simulink subsystem "ACS"  (R2025a)
settings: Solver=VariableStepAuto  StartTime=0.0  StopTime=10.0  RelTol=1e-3
settings Model: Creator=Глеб  LastModifiedBy=Глеб

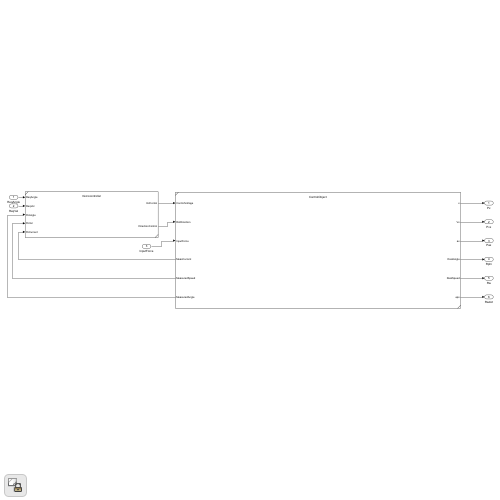
[thumbnail: Simulink's stored preview of the top-level diagram]
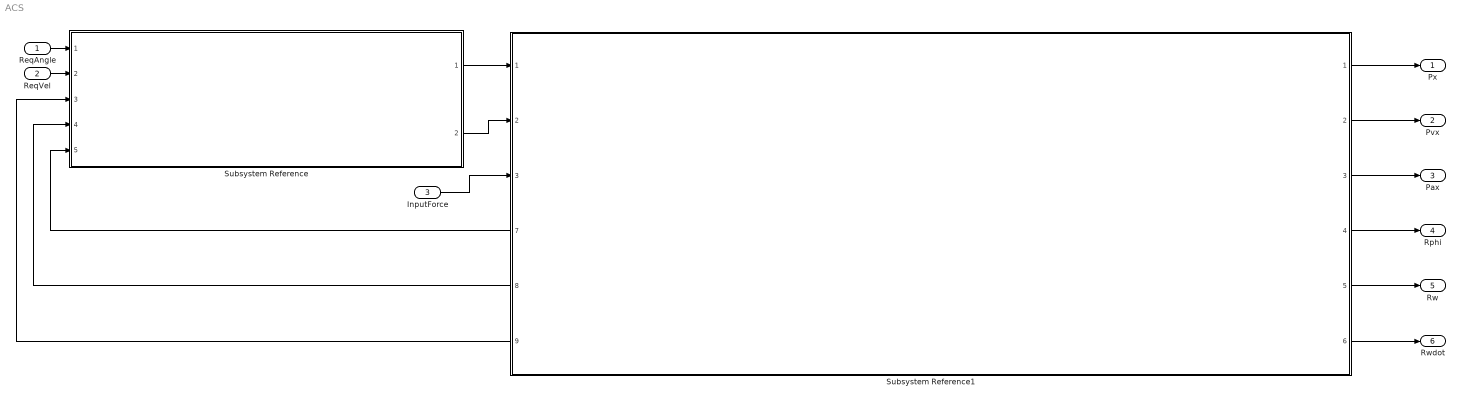
== system ACS ==
  ReqAngle : Inport
  ReqVel : Inport  Port=2
  InputForce : Inport  Port=3
  Subsystem Reference : Subsystem  ReferencedSubsystem=microcontroller
  Subsystem Reference1 : Subsystem  ReferencedSubsystem=ControlObject
      settings: PortSchema="{\"entries\":[{\"content\":{\"sides\":[{\"content\":{\"connectorIds\":[\"In1\",\"In2\",\"In3\",\"Out7\",\"Out8\",\"Out9\"]},\"type\":\"ConnectorPlacement.EquallySpacedRectSide\",\"uuid\":\"186974e8-f72a-4b37-bad7-12b1ef69ccf2\"},{\"content\":{\"connectorIds\":[\"Out1\",\"Out2\",\"Out3\",\"Out4\",\"Out5\",\"Out6\"],\"side\":\"RIGHT\"},\"type\":\"ConnectorPlacement.EquallySpacedRectSide\",\"uuid\":\"db95b573-e6f8-4acf-afcb-1eed4b262e65\"},{\"content\":{\"side\":\"TOP\"},\"type\":\"ConnectorPlacement.EquallySpacedRectSide\",\"uuid\":\"dbb95d46-234c-4790-af24-a78a943c6ee0\"}]},\"type\":\"ConnectorPlacement.EquallySpacedConnector\",\"uuid\":\"3efe73cc-2bc1-4c6d-a223-9c33f59425f8\"}],\"packageUris\":[\"http://schema.mathworks.com/mf0/Connector/R2020b\"],\"version\":\"1.0\"}"
  Px : Outport
  Pvx : Outport  Port=2
  Pax : Outport  Port=3
  Rphi : Outport  Port=4
  Rw : Outport  Port=5
  Rwdot : Outport  Port=6
  wires:
  Subsystem Reference1/3 -> Pax/1
  Subsystem Reference1/8 -> Subsystem Reference/4
  Subsystem Reference/2 -> Subsystem Reference1/2
  Subsystem Reference1/5 -> Rw/1
  Subsystem Reference1/4 -> Rphi/1
  Subsystem Reference1/9 -> Subsystem Reference/3
  Subsystem Reference1/1 -> Px/1
  Subsystem Reference1/7 -> Subsystem Reference/5
  ReqVel/1 -> Subsystem Reference/2
  InputForce/1 -> Subsystem Reference1/3
  ReqAngle/1 -> Subsystem Reference/1
  Subsystem Reference1/2 -> Pvx/1
  Subsystem Reference/1 -> Subsystem Reference1/1
  Subsystem Reference1/6 -> Rwdot/1
